simulink model "mask"  (R2020a)
settings: Solver=VariableStepAuto  StartTime=0.0  StopTime=10.0  RelTol=1e-3
settings Model: Creator=Riyansh  LastModifiedBy=Riyansh

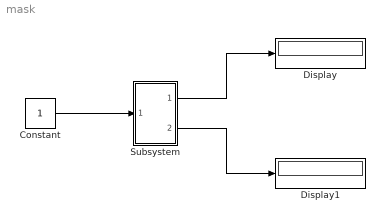
== system mask ==
  Constant : Constant
  Display : Display
  Display1 : Display
  Subsystem : Subsystem  mask{A=0, B=0}
  wires:
  Constant/1 -> Subsystem/1(In1)
  Subsystem/1(Out1) -> Display/1
  Subsystem/2(Out2) -> Display1/1

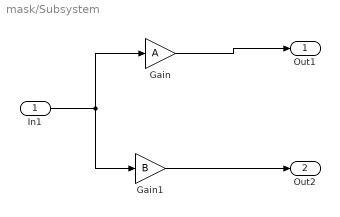
== system mask/Subsystem ==
  In1 : Inport
  Gain : Gain  Gain=A
  Gain1 : Gain  Gain=B
  Out1 : Outport
  Out2 : Outport  Port=2
  wires:
  In1/1 -> Gain1/1, Gain/1
  Gain1/1 -> Out2/1
  Gain/1 -> Out1/1
